simulink model "BLDC_220823"  (R2017a)
settings: Solver=FixedStepDiscrete  StartTime=0.0  StopTime=inf  FixedStep=0.001  RelTol=1e-3
undefined symbols (not defined in the file or in its folder): sigbuilder_block
libraries: simulink x9, GPIO_Lib x7, STM32_Config_Lib x1, TIMERS_Lib x1
settings Model: Creator=Administrator  LastModifiedBy=Administrator
settings DataIOCC: LoadExternalInput=on
settings OptimizationCC: DefaultParameterBehavior=Inlined  PassReuseOutputArgsAs=Individual arguments
settings DebuggingCC: ParameterTunabilityLossMsg=error
settings HardwareCC: ProdBitPerPointer=32  ProdBitPerSizeT=32  ProdBitPerPtrDiffT=32  ProdLargestAtomicInteger=Integer  ProdWordSize=32  ProdHWDeviceType=STMicroelectronics->STM32 32-bit Cortex-M
settings SFSimCC: MATLABDynamicMemAlloc=off
settings RTWCC: SystemTargetFile=stm32.tlc  TemplateMakefile=stm32.tmf  Description=stm32 (Embedded Target)  GenerateReport=on  IncludeHyperlinkInReport=on  GenerateTraceInfo=on  GenerateTraceReport=on  GenerateTraceReportSl=on  GenerateTraceReportSf=on  GenerateTraceReportEml=on
settings CodeAppCC: ForceParamTrailComments=on  IgnoreCustomStorageClasses=off  MaxIdLength=64  OperatorAnnotations=on  SimulinkDataObjDesc=on  SFDataObjDesc=on  MATLABFcnDesc=on  CustomSymbolStrType=$N$R$M  SimulinkBlockComments=off  MATLABSourceComments=on
settings STFCustomTargetCC: TargetLangStandard=C99 (ISO)  CodeReplacementLibrary=ARM CMSIS SIN COS  MultiwordLength=256  ParMdlRefBuildCompliant=on  IncludeMdlTerminateFcn=off  CombineOutputUpdateFcns=on  ERTCustomFileBanners=on  SupportContinuousTime=off  SupportNonInlinedSFcns=off  RemoveResetFunc=on  MATLABClassNameForMDSCustomization=Simulink.SoftwareTarget.ERTCustomization  GRTInterface=off  SystemTargetFile=stm32.tlc
settings ERTTargetCC: TargetLangStandard=C99 (ISO)  CodeReplacementLibrary=ARM CMSIS SIN COS  CompOptLevelCompliant=off  ConcurrentExecutionCompliant=off  IncludeMdlTerminateFcn=off  ERTFirstTimeCompliant=off  ModelStepFunctionPrototypeControlCompliant=off  CPPClassGenCompliant=off  UseToolchainInfoCompliant=off  ExtModeStaticAllocSize=256  ExtModeMexArgs=0,1,115200,10  InlinedParameterPlacement=NonHierarchical  ERTSrcFileBannerTemplate=sourceFileTemplate.cgt  ERTHdrFileBannerTemplate=sourceFileTemplate.cgt  ERTDataSrcFileTemplate=sourceFileTemplate.cgt  ERTDataHdrFileTemplate=sourceFileTemplate.cgt  ERTCustomFileTemplate=customRoutineProcess.tlc

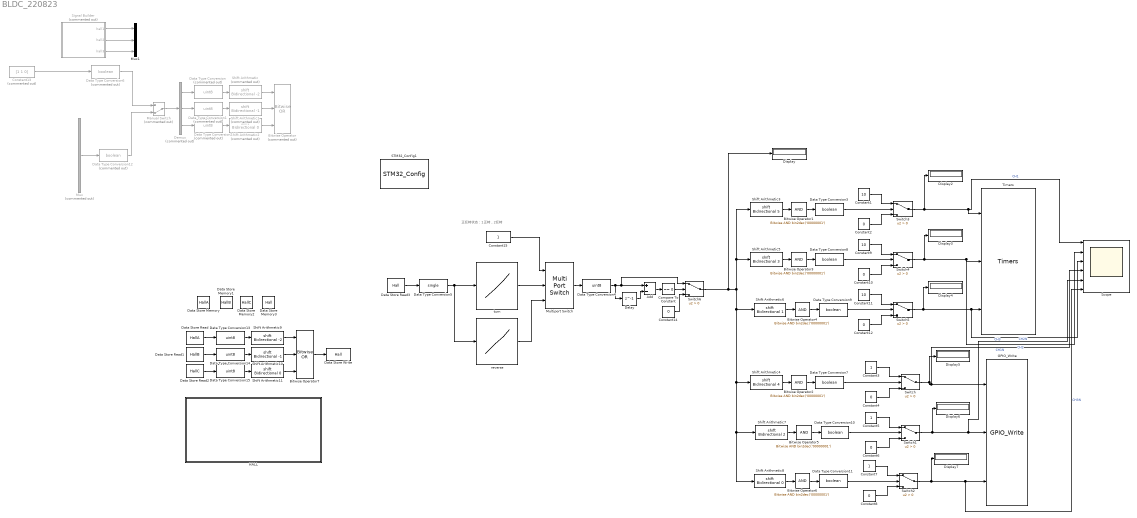
== system BLDC_220823 ==
  note: 正反转状态：1正转，2反转
  Add : Sum  Inputs=+-
  Bitwise Operator : simulink/Logic and Bit Operations/Bitwise Operator  Commented=on  logicop=OR  UseBitMask=off  NumInputPorts=3  BitMask=bin2dec('11011001')  BitMaskRealWorld=Stored Integer
  Bitwise Operator{1..6} (6 alike) : simulink/Logic and Bit Operations/Bitwise Operator  logicop=AND  UseBitMask=on  BitMask=bin2dec('00000001')  BitMaskRealWorld=Stored Integer
  Bitwise Operator7 : simulink/Logic and Bit Operations/Bitwise Operator  logicop=OR  UseBitMask=off  NumInputPorts=3  BitMask=bin2dec('11011001')  BitMaskRealWorld=Stored Integer
  Compare To Constant : simulink/Logic and Bit Operations/Compare To Constant  relop===  const=0  OutDataTypeStr=boolean
  Constant1 : Constant  Value=10
  Constant{2,4,6,8,10,12} (6 alike) : Constant  Value=0
  Constant11 : Constant  Value=10
  Constant13 : Constant  Commented=on  Value=[1 1 0]
  Constant14 : Constant  Value=0  OutDataTypeStr=uint8
  Constant{3,5,7,15} (4 alike) : Constant
  Constant9 : Constant  Value=10
  Data Store Memory : DataStoreMemory  DataStoreName=HallA  ReadBeforeWriteMsg=warning  WriteAfterWriteMsg=warning  WriteAfterReadMsg=warning  ShowAdditionalParam=off
  Data Store Memory1 : DataStoreMemory  DataStoreName=HallB  ReadBeforeWriteMsg=warning  WriteAfterWriteMsg=warning  WriteAfterReadMsg=warning  ShowAdditionalParam=off
  Data Store Memory2 : DataStoreMemory  DataStoreName=HallC  ReadBeforeWriteMsg=warning  WriteAfterWriteMsg=warning  WriteAfterReadMsg=warning  ShowAdditionalParam=off
  Data Store Memory3 : DataStoreMemory  DataStoreName=Hall  ReadBeforeWriteMsg=warning  WriteAfterWriteMsg=warning  WriteAfterReadMsg=warning  ShowAdditionalParam=off
  Data Store Read : DataStoreRead  DataStoreName=HallA
  Data Store Read1 : DataStoreRead  DataStoreName=HallB
  Data Store Read2 : DataStoreRead  DataStoreName=HallC
  Data Store Read3 : DataStoreRead  DataStoreName=Hall
  Data Store Write : DataStoreWrite  DataStoreName=Hall
  Data Type Conversion : DataTypeConversion  Commented=on  OutDataTypeStr=uint8
  Data Type Conversion1 : DataTypeConversion  Commented=on  OutDataTypeStr=uint8
  Data Type Conversion{3,7..11} (6 alike) : DataTypeConversion  OutDataTypeStr=boolean
  Data Type Conversion12 : DataTypeConversion  Commented=on  OutDataTypeStr=boolean
  Data Type Conversion{4,13..15} (4 alike) : DataTypeConversion  OutDataTypeStr=uint8
  Data Type Conversion2 : DataTypeConversion  Commented=on  OutDataTypeStr=uint8
  Data Type Conversion5 : DataTypeConversion  OutDataTypeStr=single
  Data Type Conversion6 : DataTypeConversion  Commented=on  OutDataTypeStr=boolean
  Delay : Delay  DelayLength=1  InitialCondition=0
  Demux : Demux  Commented=on  Outputs=3
  Display{,2..7} (7 alike) : Display
      settings: Format=binary (Stored Integer)
  GPIO_Write : GPIO_Lib/GPIO_Write  Port_name=GPIOB  Pin0=off  Toggle_Pin0=off  Pin1=off  Toggle_Pin1=off  Pin2=off  Toggle_Pin2=off  Pin3=off  Toggle_Pin3=off  Pin4=off  Toggle_Pin4=off  Pin5=off  Toggle_Pin5=off  Pin6=off  Toggle_Pin6=off  Pin7=off  Toggle_Pin7=off  Pin8=off  Toggle_Pin8=off  Pin9=off  Toggle_Pin9=off  Pin10=off  Toggle_Pin10=off  Pin11=off  Toggle_Pin11=off  Pin12=off  Toggle_Pin12=off  Pin13=on  Toggle_Pin13=off  Pin14=on  Toggle_Pin14=off  Pin15=on  Toggle_Pin15=off  PinList="GPIOB13  14  15"
      settings: SourceProductName=Target Support Package - STM32 Adapter
  HALL : Subsystem
  Manual Switch : ManualSwitch  Commented=on  CurrentSetting=0
  Multiport Switch : MultiPortSwitch  Inputs=2
  Mux : Mux  Commented=on  Inputs=3
  Mux1 : Mux  Inputs=3
  STM32_Config1 : STM32_Config_Lib/STM32_Config  Priority=0  Project_Path=.\  Config_File=BLDC_driver.ioc  MCU_Name=STM32F405RGTx
      settings: SourceProductName=Target Support Package - STM32 Adapter
  Scope : Scope  NumInputPorts=6
  Shift Arithmetic : ArithShift  Commented=on  BitShiftNumber=-2
  Shift Arithmetic1 : ArithShift  Commented=on  BitShiftNumber=-1
  Shift Arithmetic10 : ArithShift  BitShiftNumber=-1
  Shift Arithmetic11 : ArithShift
  Shift Arithmetic2 : ArithShift  Commented=on
  Shift Arithmetic3 : ArithShift  BitShiftNumber=5
  Shift Arithmetic4 : ArithShift  BitShiftNumber=4
  Shift Arithmetic5 : ArithShift  BitShiftNumber=3
  Shift Arithmetic6 : ArithShift  BitShiftNumber=1
  Shift Arithmetic7 : ArithShift  BitShiftNumber=2
  Shift Arithmetic8 : ArithShift
  Shift Arithmetic9 : ArithShift  BitShiftNumber=-2
  Signal Builder : Subsystem  Tag=STV Subsys  Commented=on  LoadFcn=sigbuilder_block('load');  StartFcn=sigbuilder_block('start');  StopFcn=sigbuilder_block('stop');  ClipboardFcn=sigbuilder_block('clipboard');  mask(Sigbuilder block){tuvar=[0:10]}
      mask help: Simulink:masks:SigbuilderBlock_MD
      mask init:
      | if ~strcmp(get_param(bdroot(gcbh),'SimulationStatus'),'stopped') tuvar = sigbuilder_block('maskInit'); end
      settings: CopyFcn=sigbuilder_block('copy');  DeleteFcn=sigbuilder_block('delete');  ModelCloseFcn=sigbuilder_block('modelClose');  PreSaveFcn=sigbuilder_block('preSave');  PauseFcn=sigbuilder_block('pause');  ContinueFcn=sigbuilder_block('continue');  NameChangeFcn=sigbuilder_block('namechange');  OpenFcn=sigbuilder_block('open',[56.5 41.5 543.5 352 ]);  CloseFcn=sigbuilder_block('close');
      mask Display: plot(0, 0, 100, 100,[2, 2, 32, 32, 2], [68, 8, 8, 68, 68],[32, 2], [38, 38], [32, 19, 2],[53, 60, 44], [32, 17, 17, 2],[16, 16, 31, 31]);txt = getActiveGroup(gcbh);text(2, 100, txt,'verticalAlignment', 'top');
  Switch{,1..6} (7 alike) : Switch  Criteria=u2 > Threshold
  Timers : TIMERS_Lib/Timers  currentTIM=TIM1  TIM_Name=TIM1  TIM_APBClock=168000000  TIM_Set_Clk=on  TIM_Prescaler=0  TIM_Clock=168000000.00  Variable_frequency=off  TIM_Set_OutFreq=on  TIM_ARR=8400  Output_frequency=20000.00  Repetition_counter=0  TIM_Mode=Up  TIM_DMA=none  TIM_IRQ=off  TIM_IRQ_ONLY=off  TIM_UP=off  TIM_TRG=off  TIM_COM=off  TIM_BRK=off  NbTIM=1  CH1_enable=on  CH1N_enable=off  CH1_type=Output_Comp  CH1_DMA=off  CH1_int=off  CH1_edge=Rising  CH1_div=1  CH1_variable_duty=on  CH1_set_pulse=on  CH1_output_duty=0  CH1_pulse=0  CH2_enable=on  CH2N_enable=off  CH2_type=Output_Comp  CH2_DMA=off  CH2_int=off  CH2_edge=Rising  CH2_div=1  CH2_variable_duty=on  CH2_set_pulse=on  CH2_output_duty=0  CH2_pulse=0  CH3_enable=on  CH3N_enable=off  CH3_type=Output_Comp  CH3_DMA=off  CH3_int=off  CH3_edge=Rising  CH3_div=1  CH3_variable_duty=on  CH3_set_pulse=on  CH3_output_duty=0  CH3_pulse=0  CH4_enable=off  CH4N_enable=off  CH4_type=Unknown  CH4_DMA=off  CH4_int=off  CH4_edge=Rising  CH4_div=1  CH4_variable_duty=off  CH4_set_pulse=off  CH4_output_duty=0.00  CH4_pulse=0
      settings: SourceProductName=Target Support Package - STM32 Adapter
  reverse : Lookup_n-D  NumberOfTableDimensions=1  BreakpointsForDimension1=[0 1 2 3 4 5 6 7]  Table=[0 9 36 33 18 24 6 0]  InternalRulePriority=Speed  RndMeth=Simplest  InputSameDT=on
  turn : Lookup_n-D  NumberOfTableDimensions=1  BreakpointsForDimension1=[0 1 2 3 4 5 6 7]  Table=[0 6 24 18 33 36 9 0]  InternalRulePriority=Speed  RndMeth=Simplest  InputSameDT=on
  wires:
  Constant3/1 -> Switch/1
  Constant4/1 -> Switch/3
  Constant5/1 -> Switch1/1
  Constant6/1 -> Switch1/3
  Constant8/1 -> Switch2/3
  Constant7/1 -> Switch2/1
  Switch2/1 -> Display7/1, GPIO_Write/3, Scope/6  "CH3N"
  Constant11/1 -> Switch5/1
  Constant12/1 -> Switch5/3
  Constant10/1 -> Switch4/3
  Constant9/1 -> Switch4/1
  Constant2/1 -> Switch3/3
  Constant1/1 -> Switch3/1
  Demux/1 -> Data Type Conversion/1
  Demux/2 -> Data Type Conversion1/1
  Demux/3 -> Data Type Conversion2/1
  Data Type Conversion/1 -> Shift Arithmetic/1
  Data Type Conversion1/1 -> Shift Arithmetic1/1
  Data Type Conversion2/1 -> Shift Arithmetic2/1
  Shift Arithmetic/1 -> Bitwise Operator/1
  Shift Arithmetic1/1 -> Bitwise Operator/2
  Shift Arithmetic2/1 -> Bitwise Operator/3
  Multiport Switch/1 -> Data Type Conversion4/1
  Data Type Conversion5/1 -> reverse/1, turn/1
  Shift Arithmetic3/1 -> Bitwise Operator1/1
  Data Type Conversion3/1 -> Switch3/2
  Bitwise Operator1/1 -> Data Type Conversion3/1
  Bitwise Operator2/1 -> Data Type Conversion7/1
  Shift Arithmetic4/1 -> Bitwise Operator2/1
  Data Type Conversion7/1 -> Switch/2
  Bitwise Operator3/1 -> Data Type Conversion8/1
  Shift Arithmetic5/1 -> Bitwise Operator3/1
  Data Type Conversion8/1 -> Switch4/2
  Shift Arithmetic6/1 -> Bitwise Operator4/1
  Bitwise Operator4/1 -> Data Type Conversion9/1
  Data Type Conversion9/1 -> Switch5/2
  Shift Arithmetic7/1 -> Bitwise Operator5/1
  Bitwise Operator5/1 -> Data Type Conversion10/1
  Data Type Conversion10/1 -> Switch1/2
  Bitwise Operator6/1 -> Data Type Conversion11/1
  Shift Arithmetic8/1 -> Bitwise Operator6/1
  Data Type Conversion11/1 -> Switch2/2
  Mux/1 -> Data Type Conversion12/1
  Manual Switch/1 -> Demux/1
  Data Type Conversion6/1 -> Manual Switch/1
  Data Type Conversion12/1 -> Manual Switch/2
  Add/1 -> Compare To Constant/1
  Delay/1 -> Add/2
  Compare To Constant/1 -> Switch6/2
  Constant14/1 -> Switch6/3
  Data Type Conversion4/1 -> Delay/1, Switch6/1, Add/1
  Signal Builder/1("hall1 ") -> Mux1/1
  Signal Builder/2(hall2) -> Mux1/2
  Signal Builder/3(hall3) -> Mux1/3
  Constant13/1 -> Data Type Conversion6/1
  Switch6/1 -> Display/1, Shift Arithmetic5/1, Shift Arithmetic3/1, Shift Arithmetic6/1, Shift Arithmetic4/1, Shift Arithmetic8/1, Shift Arithmetic7/1
  Switch1/1 -> Display6/1, Scope/5, GPIO_Write/2  "CH2N"
  Switch4/1 -> Display3/1, Scope/2, Timers/2  "CH2"
  Switch3/1 -> Display2/1, Scope/1, Timers/1  "CH1"
  Switch/1 -> Display5/1, Scope/4, GPIO_Write/1  "CH1N"
  Switch5/1 -> Display4/1, Scope/3, Timers/3  "CH3"
  turn/1 -> Multiport Switch/2
  reverse/1 -> Multiport Switch/3
  Constant15/1 -> Multiport Switch/1
  Bitwise Operator7/1 -> Data Store Write/1
  Shift Arithmetic11/1 -> Bitwise Operator7/3
  Shift Arithmetic10/1 -> Bitwise Operator7/2
  Shift Arithmetic9/1 -> Bitwise Operator7/1
  Data Type Conversion15/1 -> Shift Arithmetic11/1
  Data Type Conversion14/1 -> Shift Arithmetic10/1
  Data Type Conversion13/1 -> Shift Arithmetic9/1
  Data Store Read2/1 -> Data Type Conversion15/1
  Data Store Read1/1 -> Data Type Conversion14/1
  Data Store Read/1 -> Data Type Conversion13/1
  Data Store Read3/1 -> Data Type Conversion5/1

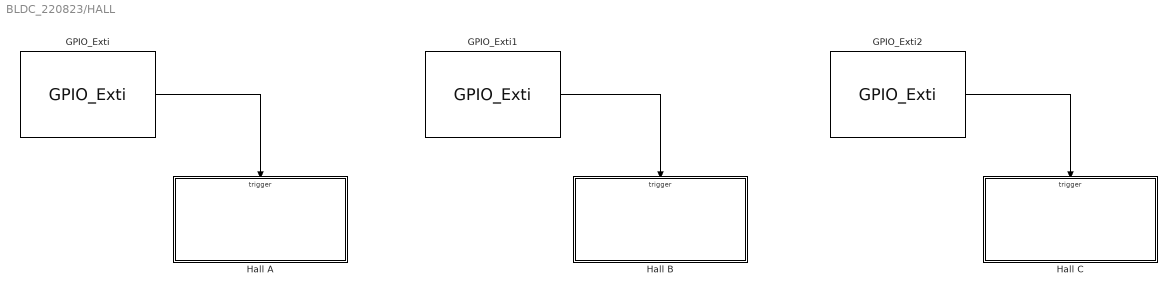
== system BLDC_220823/HALL ==
  GPIO_Exti : GPIO_Lib/GPIO_Exti  Port_name=GPIOB  Pin_0=off  Pin_1=off  Pin_2=off  Pin_3=off  Pin_4=off  Pin_5=off  Pin_6=on  Pin_7=off  Pin_8=off  Pin_9=off  Pin_10=off  Pin_11=off  Pin_12=off  Pin_13=off  Pin_14=off  Pin_15=off  PinList="GPIOB6  7  8"
      settings: SourceProductName=Target Support Package - STM32 Adapter
  GPIO_Exti1 : GPIO_Lib/GPIO_Exti  Port_name=GPIOB  Pin_0=off  Pin_1=off  Pin_2=off  Pin_3=off  Pin_4=off  Pin_5=off  Pin_6=off  Pin_7=on  Pin_8=off  Pin_9=off  Pin_10=off  Pin_11=off  Pin_12=off  Pin_13=off  Pin_14=off  Pin_15=off  PinList="GPIOB6  7  8"
      settings: SourceProductName=Target Support Package - STM32 Adapter
  GPIO_Exti2 : GPIO_Lib/GPIO_Exti  Port_name=GPIOB  Pin_0=off  Pin_1=off  Pin_2=off  Pin_3=off  Pin_4=off  Pin_5=off  Pin_6=off  Pin_7=off  Pin_8=on  Pin_9=off  Pin_10=off  Pin_11=off  Pin_12=off  Pin_13=off  Pin_14=off  Pin_15=off  PinList="GPIOB6  7  8"
      settings: SourceProductName=Target Support Package - STM32 Adapter
  Hall A : Subsystem  TreatAsAtomicUnit=on
  Hall B : Subsystem  TreatAsAtomicUnit=on
  Hall C : Subsystem  TreatAsAtomicUnit=on
  wires:
  GPIO_Exti2/1 -> Hall C/Trigger
  GPIO_Exti/1 -> Hall A/Trigger
  GPIO_Exti1/1 -> Hall B/Trigger

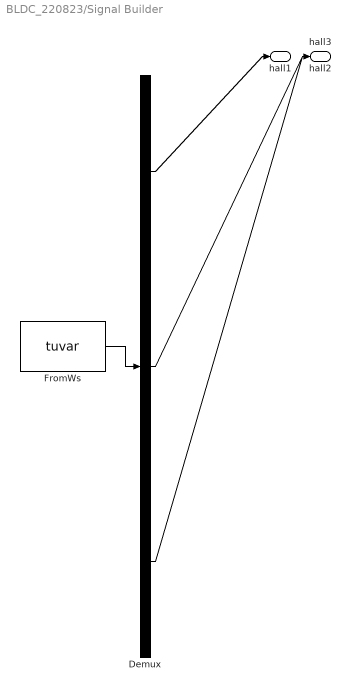
== system BLDC_220823/Signal Builder ==
  Demux : Demux  Tag=STV Demux  Outputs=3
  FromWs : FromWorkspace  Tag=STV FromWs  VariableName=tuvar  SampleTime=0
      SigBuilderData=|
      | common.afterFinalStr = 'Extrapolate'
      | common.sampleTime = 0
      | dataSet(1).timeRange = [0 10]
      | dataSet(1).name = 'Group 1'
      | dataSet(2).timeRange = [1 7]
      | dataSet(2).name = 'Sheet1'
      | sbobj.Groups(1).Name = 'Group 1'
      | sbobj.Groups(1).Signals(1).Name = 'hall1 '
      | sbobj.Groups(1).Signals(1).XData = [0 1 1.001 2 2.001 3 3.001 4 4.001 5 5.001 6 10]
      | sbobj.Groups(1).Signals(1).YData = [0 0 0 0 1 1 1 1 1 1 0 0 0]
      | sbobj.Groups(1).Signals(2).Name = 'hall2'
      | sbobj.Groups(1).Signals(2).XData = [0 1 1.001 2 2.001 3 3.001 4 4.001 5 5.001 6 6.001 10]
      | sbobj.Groups(1).Signals(2).YData = [0 0 0 0 0 0 1 1 1 1 1 1 0 0]
      | sbobj.Groups(1).Signals(3).Name = 'hall3'
      | sbobj.Groups(1).Signals(3).XData = [0 1 1.001 2 2.001 3 3.001 4 4.001 5 5.001 6 6.001 10]
      | sbobj.Groups(1).Signals(3).YData = [1 1 0 0 0 0 0 0 1 1 1 1 0 0]
      | sbobj.Groups(2).Name = 'Sheet1'
      | sbobj.Groups(2).Signals(1).Name = 'hall1 '
      | sbobj.Groups(2).Signals(1).XData = [0 1 1.001 2 2.001 3 3.001 4 4.001 5 5.001 6 10]
      | sbobj.Groups(2).Signals(1).YData = [0 0 0 0 1 1 1 1 1 1 0 0 0]
      | sbobj.Groups(2).Signals(2).Name = 'hall2'
      | sbobj.Groups(2).Signals(2).XData = [0 1 1.001 2 2.001 3 3.001 4 4.001 5 5.001 6 6.001 10]
      | sbobj.Groups(2).Signals(2).YData = [0 0 0 0 0 0 1 1 1 1 1 1 0 0]
      | sbobj.Groups(2).Signals(3).Name = 'hall3'
      | sbobj.Groups(2).Signals(3).XData = [0 1 1.001 2 2.001 3 3.001 4 4.001 5 5.001 6 6.001 10]
      | sbobj.Groups(2).Signals(3).YData = [1 1 0 0 0 0 0 0 1 1 1 1 0 0]
  "hall1 " : Outport  Tag=STV Outport
  hall2 : Outport  Tag=STV Outport  Port=2
  hall3 : Outport  Tag=STV Outport  Port=3
  wires:
  FromWs/1 -> Demux/1
  Demux/1 -> "hall1 "/1
  Demux/2 -> hall2/1
  Demux/3 -> hall3/1

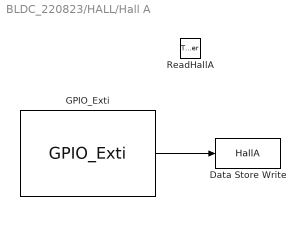
== system BLDC_220823/HALL/Hall A ==
  ReadHallA : TriggerPort  TriggerType=function-call  VariantControl=Variant
  Data Store Write : DataStoreWrite  DataStoreName=HallA
  GPIO_Exti : GPIO_Lib/GPIO_Exti  Port_name=GPIOB  Pin_0=off  Pin_1=off  Pin_2=off  Pin_3=off  Pin_4=off  Pin_5=off  Pin_6=on  Pin_7=off  Pin_8=off  Pin_9=off  Pin_10=off  Pin_11=off  Pin_12=off  Pin_13=off  Pin_14=off  Pin_15=off  PinList="GPIOB6  7  8"
      settings: SourceProductName=Target Support Package - STM32 Adapter
  wires:
  GPIO_Exti/1 -> Data Store Write/1

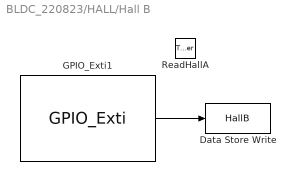
== system BLDC_220823/HALL/Hall B ==
  ReadHallA : TriggerPort  TriggerType=function-call  VariantControl=Variant
  Data Store Write : DataStoreWrite  DataStoreName=HallB
  GPIO_Exti1 : GPIO_Lib/GPIO_Exti  Port_name=GPIOB  Pin_0=off  Pin_1=off  Pin_2=off  Pin_3=off  Pin_4=off  Pin_5=off  Pin_6=off  Pin_7=on  Pin_8=off  Pin_9=off  Pin_10=off  Pin_11=off  Pin_12=off  Pin_13=off  Pin_14=off  Pin_15=off  PinList="GPIOB6  7  8"
      settings: SourceProductName=Target Support Package - STM32 Adapter
  wires:
  GPIO_Exti1/1 -> Data Store Write/1

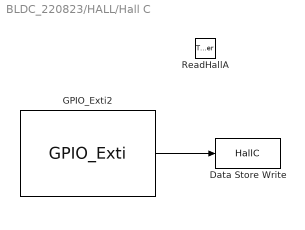
== system BLDC_220823/HALL/Hall C ==
  ReadHallA : TriggerPort  TriggerType=function-call  VariantControl=Variant
  Data Store Write : DataStoreWrite  DataStoreName=HallC
  GPIO_Exti2 : GPIO_Lib/GPIO_Exti  Port_name=GPIOB  Pin_0=off  Pin_1=off  Pin_2=off  Pin_3=off  Pin_4=off  Pin_5=off  Pin_6=off  Pin_7=off  Pin_8=on  Pin_9=off  Pin_10=off  Pin_11=off  Pin_12=off  Pin_13=off  Pin_14=off  Pin_15=off  PinList="GPIOB6  7  8"
      settings: SourceProductName=Target Support Package - STM32 Adapter
  wires:
  GPIO_Exti2/1 -> Data Store Write/1
